simulink model "manipJointTrajectory"  (R2021a)
settings: Solver=FixedStepAuto  StartTime=0.0  StopTime=inf  RelTol=1e-3
PreLoadFcn:
  | createWaypointData;
undefined symbols (not defined in the file): diff, gen3, jointAnglesHome, maxWaypoints, numJoints, ts, waypointTimes
libraries: trajExampleUtils x9, robotcorelib x3, robotmaniplib x2
settings Model: Creator=scastro  LastModifiedBy=dzy
settings SolverCC: AlgebraicLoopSolver=TrustRegion
settings DataIOCC: ReturnWorkspaceOutputs=off
settings OptimizationCC: DefaultParameterBehavior=Inlined  EnhancedBackFolding=on  PassReuseOutputArgsAs=Individual arguments  OptimizeBlockOrder=speed  DifferentSizesBufferReuse=on  OptimizationCustomize=off  EfficientTunableParamExpr=on
settings DebuggingCC: ParameterTunabilityLossMsg=error  SFMachineParentedDataDiag=warning  ArithmeticOperatorsInVariantConditions=warning
settings SFSimCC: CustomCodeUndefinedFunction=UseInterfaceOnly
settings RTWCC: SystemTargetFile=ert.tlc  TemplateMakefile=ert_default_tmf  GenerateReport=on  IncludeHyperlinkInReport=on  LaunchReport=on  GenerateTraceInfo=on  GenerateTraceReport=on  GenerateTraceReportSl=on  GenerateTraceReportSf=on  GenerateTraceReportEml=on
settings CodeAppCC: ForceParamTrailComments=on  IgnoreCustomStorageClasses=off  OperatorAnnotations=on  SimulinkDataObjDesc=on  SFDataObjDesc=on  InsertBlockDesc=on
settings ERTTargetCC: TargetLangStandard=C99 (ISO)  GenerateSampleERTMain=on  SupportVariableSizeSignals=on  InlinedParameterPlacement=NonHierarchical  ERTCustomFileTemplate=example_file_process.tlc

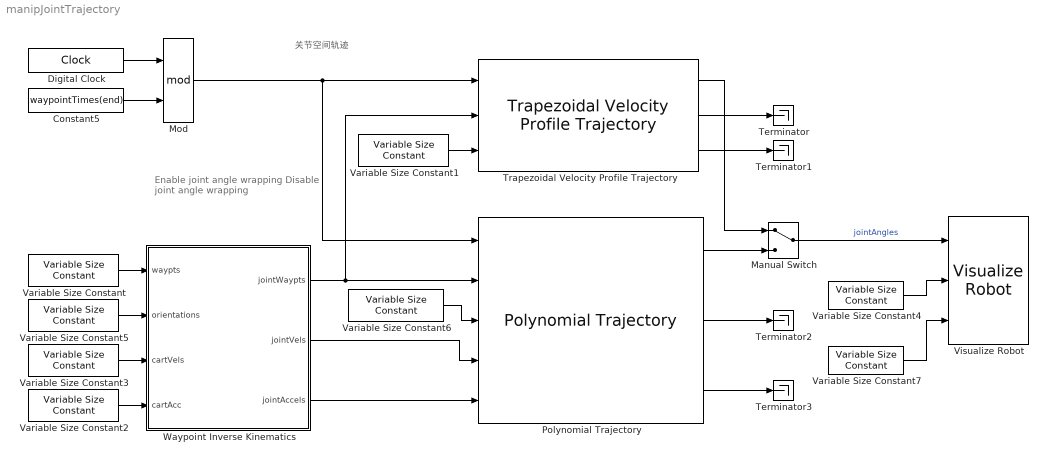
== system manipJointTrajectory ==
  note: Enable joint angle wrapping
      |
      | Disable joint angle wrapping
  note: 关节空间轨迹
  Constant5 : Constant  Value=waypointTimes(end)
  Digital Clock : DigitalClock  SampleTime=ts
  Manual Switch : ManualSwitch
  Mod : Math  Operator=mod  SignedPower=on  SaturateOnIntegerOverflow=on
  Polynomial Trajectory : robotcorelib/Polynomial Trajectory  WaypointSource=External  Waypoints=[ 0, 2, 1, 5, 0; -1, 3, 1, 4, 4 ]  TimePoints=[ 0, 1, 2, 3, 4 ]  TimeInterval=[ 1, 4 ]  Method=Quintic Polynomial  ParameterSource=External  VelocityBoundaryCondition=zeros( 2, 5 )  AccelerationBoundaryCondition=zeros( 2, 5 )  SimulateUsing=Interpreted execution
  Terminator{,1..3} (4 alike) : Terminator
  Trapezoidal Velocity Profile Trajectory : robotcorelib/Trapezoidal Velocity Profile Trajectory  WaypointSource=External  Waypoints=[ 0, -0.5, -1; 0, 0.5, 1 ]  NumParams=1  Parameter1=End Time  Parameter2=End Time  ParameterSource=External  PeakVelocity=[ 2; 2 ]  Acceleration=[ 1; 2 ]  EndTime=[ 1; 1 ]  AccelTime=[ 1; 2 ]  SimulateUsing=Interpreted execution
      settings: SourceProductBaseCode=NV,RO,RR,UV
  Variable Size Constant : trajExampleUtils/Variable Size Constant  val=waypoints  maxSize=[3,maxWaypoints]  Ts=-1
  Variable Size Constant1 : trajExampleUtils/Variable Size Constant  val=repmat(diff(waypointTimes),[numJoints 1])  maxSize=[numJoints,maxWaypoints-1]  Ts=-1
  Variable Size Constant2 : trajExampleUtils/Variable Size Constant  val=waypointAccels  maxSize=[3,maxWaypoints]  Ts=-1
  Variable Size Constant3 : trajExampleUtils/Variable Size Constant  val=waypointVels  maxSize=[3,maxWaypoints]  Ts=-1
  Variable Size Constant4 : trajExampleUtils/Variable Size Constant  val=waypoints  maxSize=[3,maxWaypoints]  Ts=-1
  Variable Size Constant5 : trajExampleUtils/Variable Size Constant  val=orientations  maxSize=[3,maxWaypoints]  Ts=-1
  Variable Size Constant6 : trajExampleUtils/Variable Size Constant  val=waypointTimes  maxSize=[1,maxWaypoints]  Ts=-1
  Variable Size Constant7 : trajExampleUtils/Variable Size Constant  val=orientations  maxSize=[3,maxWaypoints]  Ts=-1
  Visualize Robot : trajExampleUtils/Visualize Robot  rbtName=gen3  eeName=Gripper  numJoints=numel(gen3.homeConfiguration)  maxPts=maxWaypoints  plotMode=Trajectory
  Waypoint Inverse Kinematics : Subsystem  TreatAsAtomicUnit=on
  wires:
  Digital Clock/1 -> Mod/1
  Polynomial Trajectory/1 -> Manual Switch/2
  Mod/1 -> Trapezoidal Velocity Profile Trajectory/1, Polynomial Trajectory/1
  Constant5/1 -> Mod/2
  Manual Switch/1 -> Visualize Robot/1  "jointAngles"
  Variable Size Constant4/1 -> Visualize Robot/2
  Variable Size Constant/1 -> Waypoint Inverse Kinematics/1(waypts)
  Variable Size Constant6/1 -> Polynomial Trajectory/3
  Waypoint Inverse Kinematics/2(jointVels) -> Polynomial Trajectory/4
  Waypoint Inverse Kinematics/3(jointAccels) -> Polynomial Trajectory/5
  Waypoint Inverse Kinematics/1(jointWaypts) -> Polynomial Trajectory/2, Trapezoidal Velocity Profile Trajectory/2
  Variable Size Constant5/1 -> Waypoint Inverse Kinematics/2(orientations)
  Trapezoidal Velocity Profile Trajectory/1 -> Manual Switch/1
  Variable Size Constant1/1 -> Trapezoidal Velocity Profile Trajectory/3
  Trapezoidal Velocity Profile Trajectory/2 -> Terminator/1
  Trapezoidal Velocity Profile Trajectory/3 -> Terminator1/1
  Polynomial Trajectory/2 -> Terminator2/1
  Polynomial Trajectory/3 -> Terminator3/1
  Variable Size Constant3/1 -> Waypoint Inverse Kinematics/3(cartVels)
  Variable Size Constant2/1 -> Waypoint Inverse Kinematics/4(cartAcc)
  Variable Size Constant7/1 -> Visualize Robot/3

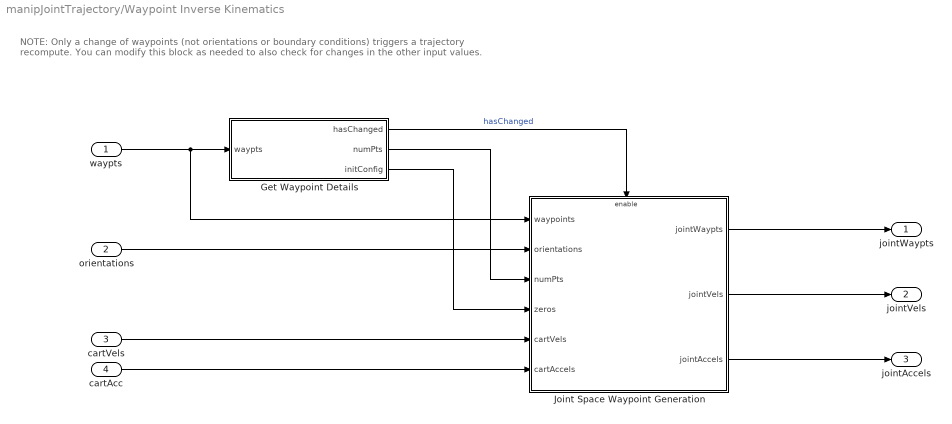
== system manipJointTrajectory/Waypoint Inverse Kinematics ==
  note: NOTE: Only a change of waypoints (not orientations or boundary conditions) triggers a trajectory recompute.
      | You can modify this block as needed to also check for changes in the other input values.
  waypts : Inport
  orientations : Inport  Port=2
  cartVels : Inport  Port=3
  cartAcc : Inport  Port=4
  Get Waypoint Details : MATLAB Function  TreatAsAtomicUnit=on
  Joint Space Waypoint Generation : Subsystem
  jointWaypts : Outport  PortDimensions=[numJoints maxWaypoints]  VectorParamsAs1DForOutWhenUnconnected=off
      settings: VarSizeSig=Yes
  jointVels : Outport  Port=2  PortDimensions=[numJoints maxWaypoints]  VectorParamsAs1DForOutWhenUnconnected=off
      settings: VarSizeSig=Yes
  jointAccels : Outport  Port=3  PortDimensions=[numJoints maxWaypoints]  VectorParamsAs1DForOutWhenUnconnected=off
      settings: VarSizeSig=Yes
  wires:
  waypts/1 -> Joint Space Waypoint Generation/1(waypoints), Get Waypoint Details/1(waypts)
  Get Waypoint Details/2(numPts) -> Joint Space Waypoint Generation/3(numPts)
  Get Waypoint Details/3(initConfig) -> Joint Space Waypoint Generation/4(zeros)
  cartVels/1 -> Joint Space Waypoint Generation/5(cartVels)
  cartAcc/1 -> Joint Space Waypoint Generation/6(cartAccels)
  Joint Space Waypoint Generation/1(jointWaypts) -> jointWaypts/1
  Joint Space Waypoint Generation/2(jointVels) -> jointVels/1
  Joint Space Waypoint Generation/3(jointAccels) -> jointAccels/1
  Get Waypoint Details/1(hasChanged) -> Joint Space Waypoint Generation/Enable  "hasChanged"
  orientations/1 -> Joint Space Waypoint Generation/2(orientations)

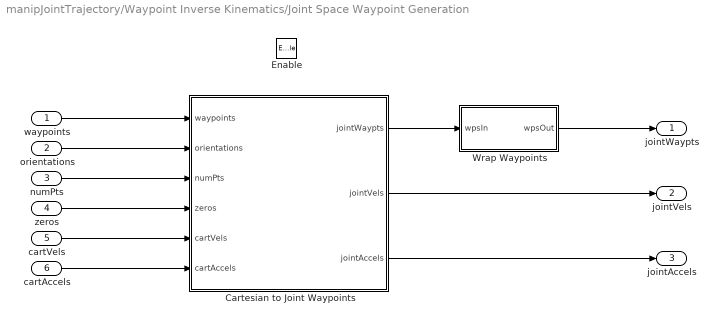
== system manipJointTrajectory/Waypoint Inverse Kinematics/Joint Space Waypoint Generation ==
  waypoints : Inport
  orientations : Inport  Port=2
  numPts : Inport  Port=3
  zeros : Inport  Port=4
  cartVels : Inport  Port=5
  cartAccels : Inport  Port=6
  Enable : EnablePort  PropagateVarSize=During execution
  Cartesian to Joint Waypoints : Subsystem
  Wrap Waypoints : MATLAB Function  TreatAsAtomicUnit=on
  jointWaypts : Outport  VectorParamsAs1DForOutWhenUnconnected=off
  jointVels : Outport  Port=2  VectorParamsAs1DForOutWhenUnconnected=off
  jointAccels : Outport  Port=3  VectorParamsAs1DForOutWhenUnconnected=off
  wires:
  Cartesian to Joint Waypoints/2(jointVels) -> jointVels/1
  Cartesian to Joint Waypoints/3(jointAccels) -> jointAccels/1
  zeros/1 -> Cartesian to Joint Waypoints/4(zeros)
  numPts/1 -> Cartesian to Joint Waypoints/3(numPts)
  Cartesian to Joint Waypoints/1(jointWaypts) -> Wrap Waypoints/1(wpsIn)
  cartAccels/1 -> Cartesian to Joint Waypoints/6(cartAccels)
  cartVels/1 -> Cartesian to Joint Waypoints/5(cartVels)
  waypoints/1 -> Cartesian to Joint Waypoints/1(waypoints)
  orientations/1 -> Cartesian to Joint Waypoints/2(orientations)
  Wrap Waypoints/1(wpsOut) -> jointWaypts/1

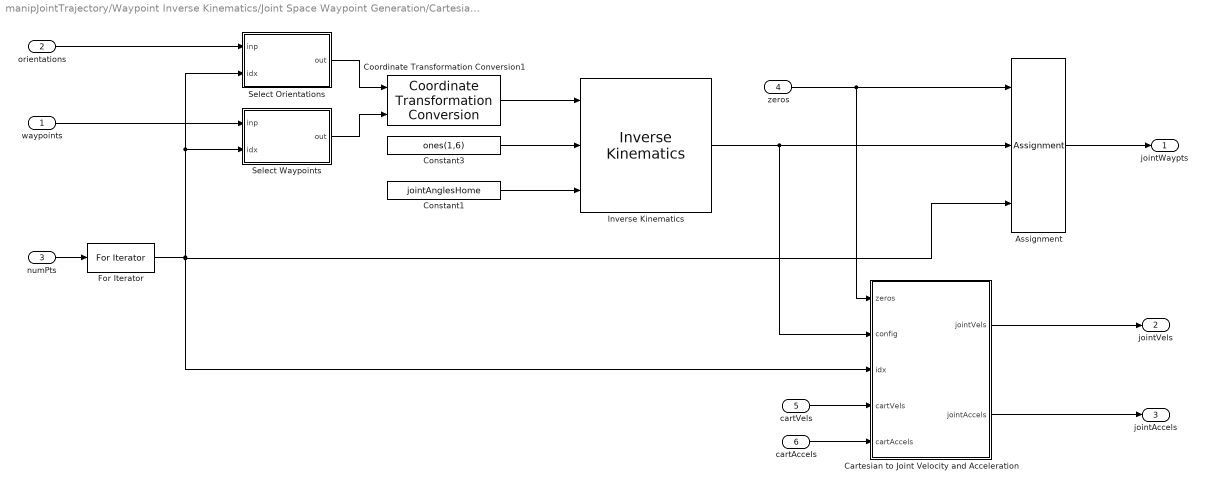
== system manipJointTrajectory/Waypoint Inverse Kinematics/Joint Space Waypoint Generation/Cartesian to Joint Waypoints ==
  waypoints : Inport
  orientations : Inport  Port=2
  numPts : Inport  Port=3
  zeros : Inport  Port=4
  cartVels : Inport  Port=5
  cartAccels : Inport  Port=6
  Assignment : Assignment  NumberOfDimensions=2  DiagnosticForDimensions=Warning  IndexOptions=Index vector (dialog),Index vector (port)  Indices=1:numJoints,1  OutputSizes=10,20
  Cartesian to Joint Velocity and Acceleration : Subsystem
  Constant1 : Constant  Value=jointAnglesHome  VectorParams1D=off
  Constant3 : Constant  Value=ones(1,6)  VectorParams1D=off
  Coordinate Transformation Conversion1 : robotcorelib/Coordinate Transformation Conversion  InputRepresentation=Euler Angles  InputEulerSequence=ZYX  ShowTrVecInputPort=on  OutputRepresentation=Homogeneous Transformation  OutputEulerSequence=ZYX  ShowTrVecOutputPort=on  SimulateUsing=Interpreted execution
      settings: SourceProductBaseCode=NV,RO,RR,UV
  For Iterator : ForIterator  ResetStates=reset  IterationSource=external
  Inverse Kinematics : robotmaniplib/Inverse Kinematics  RigidBodyTree=gen3  EndEffector=Gripper  ShowInfo=off  SolverName=BFGS Gradient Projection  EnforceJointLimits=on  MaxIterations=1500  MaxTime=10  GradientTolerance=1e-7  SolutionTolerance=1e-6  StepTolerance=1e-14  ErrorChangeTolerance=1e-12  UseErrorDamping=on  DampingBias=0.0025  SimulateUsing=Interpreted execution
  Select Orientations : MATLAB Function  TreatAsAtomicUnit=on
  Select Waypoints : MATLAB Function  TreatAsAtomicUnit=on
  jointWaypts : Outport  VectorParamsAs1DForOutWhenUnconnected=off
  jointVels : Outport  Port=2  VectorParamsAs1DForOutWhenUnconnected=off
  jointAccels : Outport  Port=3  VectorParamsAs1DForOutWhenUnconnected=off
  wires:
  zeros/1 -> Assignment/1, Cartesian to Joint Velocity and Acceleration/1(zeros)
  For Iterator/1 -> Select Orientations/2(idx), Select Waypoints/2(idx), Cartesian to Joint Velocity and Acceleration/3(idx), Assignment/3
  Assignment/1 -> jointWaypts/1
  numPts/1 -> For Iterator/1
  waypoints/1 -> Select Waypoints/1(inp)
  orientations/1 -> Select Orientations/1(inp)
  Inverse Kinematics/1 -> Cartesian to Joint Velocity and Acceleration/2(config), Assignment/2
  Coordinate Transformation Conversion1/1 -> Inverse Kinematics/1
  Constant3/1 -> Inverse Kinematics/2
  Select Orientations/1(out) -> Coordinate Transformation Conversion1/1
  Select Waypoints/1(out) -> Coordinate Transformation Conversion1/2
  cartVels/1 -> Cartesian to Joint Velocity and Acceleration/4(cartVels)
  cartAccels/1 -> Cartesian to Joint Velocity and Acceleration/5(cartAccels)
  Cartesian to Joint Velocity and Acceleration/1(jointVels) -> jointVels/1
  Cartesian to Joint Velocity and Acceleration/2(jointAccels) -> jointAccels/1
  Constant1/1 -> Inverse Kinematics/3

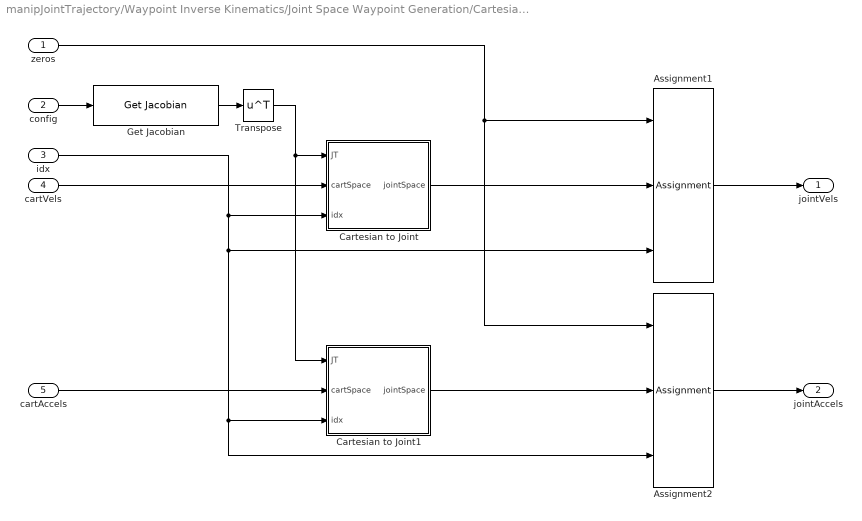
== system manipJointTrajectory/Waypoint Inverse Kinematics/Joint Space Waypoint Generation/Cartesian to Joint Waypoints/Cartesian to Joint Velocity and Acceleration ==
  zeros : Inport
  config : Inport  Port=2
  idx : Inport  Port=3
  cartVels : Inport  Port=4
  cartAccels : Inport  Port=5
  Assignment1 : Assignment  NumberOfDimensions=2  DiagnosticForDimensions=Warning  IndexOptions=Index vector (dialog),Index vector (port)  Indices=1:numJoints,1  OutputSizes=10,20
  Assignment2 : Assignment  NumberOfDimensions=2  DiagnosticForDimensions=Warning  IndexOptions=Index vector (dialog),Index vector (port)  Indices=1:numJoints,1  OutputSizes=10,20
  Cartesian to Joint : Subsystem
  Cartesian to Joint1 : Subsystem
  Get Jacobian : robotmaniplib/Get Jacobian  RigidBodyTree=gen3  EndEffector=Gripper  SimulateUsing=Interpreted execution
      settings: SourceProductBaseCode=RO
  Transpose : Math  Operator=transpose  SignedPower=on  SaturateOnIntegerOverflow=on
  jointVels : Outport  VectorParamsAs1DForOutWhenUnconnected=off
  jointAccels : Outport  Port=2  VectorParamsAs1DForOutWhenUnconnected=off
  wires:
  cartVels/1 -> Cartesian to Joint/2(cartSpace)
  zeros/1 -> Assignment2/1, Assignment1/1
  Cartesian to Joint/1(jointSpace) -> Assignment1/2
  Cartesian to Joint1/1(jointSpace) -> Assignment2/2
  Transpose/1 -> Cartesian to Joint/1(JT), Cartesian to Joint1/1(JT)
  idx/1 -> Cartesian to Joint/3(idx), Assignment2/3, Cartesian to Joint1/3(idx), Assignment1/3
  Assignment1/1 -> jointVels/1
  Get Jacobian/1 -> Transpose/1
  cartAccels/1 -> Cartesian to Joint1/2(cartSpace)
  Assignment2/1 -> jointAccels/1
  config/1 -> Get Jacobian/1

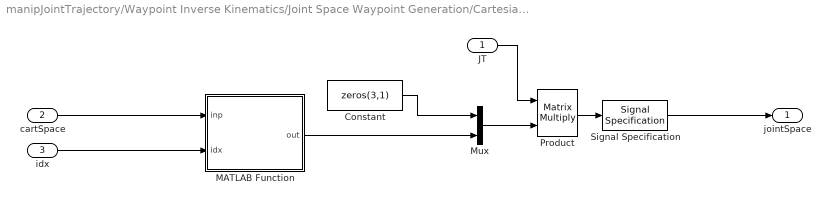
== system manipJointTrajectory/Waypoint Inverse Kinematics/Joint Space Waypoint Generation/Cartesian to Joint Waypoints/Cartesian to Joint Velocity and Acceleration/Cartesian to Joint ==
  JT : Inport
  cartSpace : Inport  Port=2
  idx : Inport  Port=3
  Constant : Constant  Value=zeros(3,1)
  MATLAB Function : MATLAB Function  TreatAsAtomicUnit=on
  Mux : Mux  Inputs=2
  Product : Product  Multiplication=Matrix(*)
  Signal Specification : SignalSpecification  Dimensions=[numJoints 1]
  jointSpace : Outport  VectorParamsAs1DForOutWhenUnconnected=off
  wires:
  Mux/1 -> Product/2
  Constant/1 -> Mux/1
  cartSpace/1 -> MATLAB Function/1(inp)
  Signal Specification/1 -> jointSpace/1
  idx/1 -> MATLAB Function/2(idx)
  Product/1 -> Signal Specification/1
  JT/1 -> Product/1
  MATLAB Function/1(out) -> Mux/2

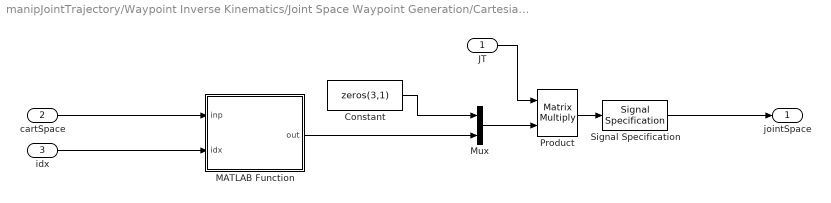
== system manipJointTrajectory/Waypoint Inverse Kinematics/Joint Space Waypoint Generation/Cartesian to Joint Waypoints/Cartesian to Joint Velocity and Acceleration/Cartesian to Joint1 ==
  JT : Inport
  cartSpace : Inport  Port=2
  idx : Inport  Port=3
  Constant : Constant  Value=zeros(3,1)
  MATLAB Function : MATLAB Function  TreatAsAtomicUnit=on
  Mux : Mux  Inputs=2
  Product : Product  Multiplication=Matrix(*)
  Signal Specification : SignalSpecification  Dimensions=[numJoints 1]
  jointSpace : Outport  VectorParamsAs1DForOutWhenUnconnected=off
  wires:
  MATLAB Function/1(out) -> Mux/2
  JT/1 -> Product/1
  Product/1 -> Signal Specification/1
  idx/1 -> MATLAB Function/2(idx)
  Signal Specification/1 -> jointSpace/1
  cartSpace/1 -> MATLAB Function/1(inp)
  Constant/1 -> Mux/1
  Mux/1 -> Product/2

== matlab function manipJointTrajectory/Waypoint Inverse Kinematics/Joint Space Waypoint Generation/Wrap Waypoints ==
  data: wpsIn input; wpsOut output size=[numJoints maxWaypoints]
function wpsOut = wrap(wpsIn)
% Prevents successive waypoints from going in the "wrong" direction by
% adding/subtracting a full revolution (2*pi) from the joint angles as
% needed.

wpsOut = wpsIn;

% Loop through successive waypoints
for wpIdx = 2:size(wpsIn,2)
    % Loop through joint angles
    for jIdx = 1:size(wpsIn,1)
        % Add/remove 2*pi radians if the difference is greater than pi
        angleDiff = diff(wpsOut(jIdx,wpIdx-1:wpIdx));
        if angleDiff > pi
            wpsOut(jIdx,wpIdx) = wpsOut(jIdx,wpIdx) - 2*pi;
        elseif angleDiff < -pi
            wpsOut(jIdx,wpIdx) = wpsOut(jIdx,wpIdx) + 2*pi;
        end
    end
    
end

== matlab function manipJointTrajectory/Waypoint Inverse Kinematics/Joint Space Waypoint Generation/Cartesian to Joint Waypoints/Cartesian to Joint Velocity and Acceleration/Cartesian to Joint/MATLAB Function ==
  data: inp input; out output size=3; idx input
function out = select(inp, idx)

% assert(numel(idx)==1)

out = inp(1:3,idx);

== matlab function manipJointTrajectory/Waypoint Inverse Kinematics/Joint Space Waypoint Generation/Cartesian to Joint Waypoints/Cartesian to Joint Velocity and Acceleration/Cartesian to Joint1/MATLAB Function ==
  data: inp input; out output size=3; idx input
function out = select(inp, idx)

% assert(numel(idx)==1)

out = inp(1:3,idx);

== matlab function manipJointTrajectory/Waypoint Inverse Kinematics/Joint Space Waypoint Generation/Cartesian to Joint Waypoints/Select Waypoints ==
  data: inp input; out output size=3; idx input
function out = select(inp, idx)

% assert(numel(idx)==1)

out = inp(1:3,idx);

== matlab function manipJointTrajectory/Waypoint Inverse Kinematics/Joint Space Waypoint Generation/Cartesian to Joint Waypoints/Select Orientations ==
  data: inp input; out output size=3; idx input
function out = select(inp, idx)

% assert(numel(idx)==1)

out = inp(1:3,idx);

== matlab function manipJointTrajectory/Waypoint Inverse Kinematics/Get Waypoint Details ==
  data: hasChanged output; waypts input; numPts output; initConfig output size=[numJoints maxWaypoints]; numJoints parameter; maxWaypoints parameter
function [hasChanged,numPts,initConfig] = getWaypointDetails(waypts,numJoints, maxWaypoints)

% Check if the waypoints or orientations have changed
persistent prevWaypts
coder.varsize('prevWaypts',[3 maxWaypoints]);
if isempty(prevWaypts)
    prevWaypts = zeros(3,maxWaypoints);
end

% Get the size of the input waypoints and output zeros of that size for
% assigning joint angles
numPts = size(waypts,2);
initConfig = zeros(numJoints,numPts);

% Check if the waypoints have changed to trigger recomputation of the
% trajectory
if isequal(prevWaypts,waypts)
    hasChanged = false;
else
    hasChanged = true;
    prevWaypts = waypts;
end
